simulink model "ejh44b"  (Simulink 3.00)
settings: Solver=ode45  StartTime=0.0  StopTime=10.0  RelTol=1e-3
settings Model: LastModifiedBy=Administrador

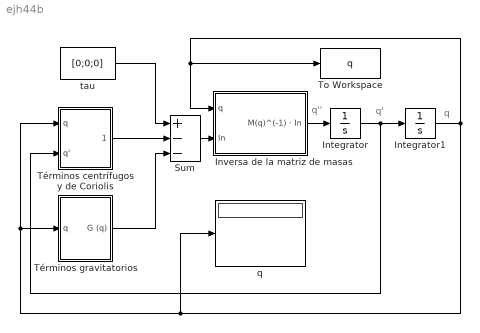
== system ejh44b ==
  note: q'
  note: q''
  note: q
  Integrator : Integrator  ExternalReset=none  InitialConditionSource=internal  InitialCondition=[0;0;0]  LimitOutput=off  UpperSaturationLimit=inf  LowerSaturationLimit=-inf  ShowSaturationPort=off  ShowStatePort=off  AbsoluteTolerance=auto
  Integrator1 : Integrator  ExternalReset=none  InitialConditionSource=internal  InitialCondition=[pi/6; pi/6; pi/18]  LimitOutput=off  UpperSaturationLimit=inf  LowerSaturationLimit=-inf  ShowSaturationPort=off  ShowStatePort=off  AbsoluteTolerance=auto
  Inversa de la matriz de masas : Subsystem  mask(Término de Coriolis){dyn=[0 0 0 0 0 4.7 0.8 0 0 0 0 0 0 0 0 0 1 0 0 0;0 0.8 0 0 0 2.6 0.8 0 0 0 0 0 0 0 0 0 1 0 0 0;0 0.8 0 0 0 1.1 0 0 0 0.05 0.1 0.1 0 0 0 0 1 0 0 0]}
      mask prompts: dyn "Matriz de parámetros dinámicos:"
      mask help: Este bloque devuelve el par correspondiente al término de Coriolis.
      mask Help: A este bloque hay que darle tres parámetros: 1) La matriz de parámetros dinámicos del manipulador de acuerdo con el formato que se explica en la sección "dyn" del Apéndice, 2) Un vector columna correspondiente a la aceleración de la gravedad, y 3) Un vector columna correspondiente a las fuerzas externas.
  Sum : Sum  Inputs=+--  SaturateOnIntegerOverflow=on
  To Workspace : ToWorkspace  VariableName=q  SampleTime=-1  SaveFormat=Matrix
  Términos gravitatorios : Subsystem  mask(Término gravitatorio){dyn=[0 0 0 0 0 4.7 0.8 0 0 0 0 0 0 0 0 0 1 0 0 0;0 0.8 0 0 0 2.6 0.8 0 0 0 0 0 0 0 0 0 1 0 0 0;0 0.8 0 0 0 1.1 0 0 0 0.05 0.1 0.1 0 0 0 0 1 0 0 0], grav=[0 -9.8 0]}
      mask prompts: dyn "Matriz de parámetros cinemáticos y dinámicos:"; grav "Vector aceleración de la gravedad:"
      mask help: Este bloque calcula el par correspondiente al término gravitatorio.
  Términos centrífugos y de Coriolis : Subsystem  mask(Término de Coriolis){dyn=[0 0 0 0 0 4.7 0.8 0 0 0 0 0 0 0 0 0 1 0 0 0;0 0.8 0 0 0 2.6 0.8 0 0 0 0 0 0 0 0 0 1 0 0 0;0 0.8 0 0 0 1.1 0 0 0 0.05 0.1 0.1 0 0 0 0 1 0 0 0]}
      mask prompts: dyn "Matriz de parámetros dinámicos:"
      mask help: Este bloque devuelve el par correspondiente al término de Coriolis.
      mask Help: A este bloque hay que darle tres parámetros: 1) La matriz de parámetros dinámicos del manipulador de acuerdo con el formato que se explica en la sección "dyn" del Apéndice, 2) Un vector columna correspondiente a la aceleración de la gravedad, y 3) Un vector columna correspondiente a las fuerzas externas.
  q : Display
      settings: Format=short
  tau : Constant  Value=[0;0;0]
  wires:
  Términos centrífugos y de Coriolis/1(V (q,q')) -> Sum/2
  Sum/1 -> Inversa de la matriz de masas/2(In)
  Inversa de la matriz de masas/1(M(q)^(-1) · In) -> Integrator/1
  Integrator/1 -> Integrator1/1, Términos centrífugos y de Coriolis/2(q')
  Integrator1/1 -> Inversa de la matriz de masas/1(q), To Workspace/1, Términos centrífugos y de Coriolis/1(q), Términos gravitatorios/1(q), q/1
  Términos gravitatorios/1(G (q)) -> Sum/3
  tau/1 -> Sum/1

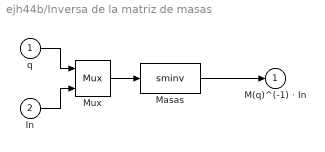
== system ejh44b/Inversa de la matriz de masas ==
  q : Inport  Port=1  PortWidth=-1  SampleTime=-1  DataType=auto
      settings: SignalType=auto
  In : Inport  Port=2  PortWidth=-1  SampleTime=-1  DataType=auto
      settings: SignalType=auto
  Masas : S-Function  FunctionName=sminv  Parameters=dyn  PortCounts=[]  SFunctionModules=''
  Mux : Mux  Inputs=2
      settings: DisplayOption=none
  M(q)^(-1) · In : Outport  Port=1  InitialOutput=0
  wires:
  Masas/1 -> M(q)^(-1) · In/1
  In/1 -> Mux/2
  q/1 -> Mux/1
  Mux/1 -> Masas/1

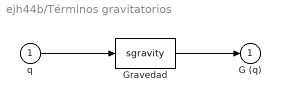
== system ejh44b/Términos gravitatorios ==
  q : Inport  Port=1  PortWidth=-1  SampleTime=-1  DataType=auto
      settings: SignalType=auto
  Gravedad : S-Function  FunctionName=sgravity  Parameters=dyn,grav  PortCounts=[]  SFunctionModules=''
  G (q) : Outport  Port=1  InitialOutput=0
  wires:
  q/1 -> Gravedad/1
  Gravedad/1 -> G (q)/1

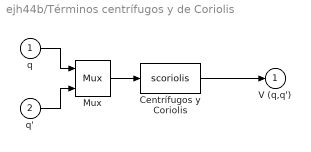
== system ejh44b/Términos centrífugos y de Coriolis ==
  q : Inport  Port=1  PortWidth=-1  SampleTime=-1  DataType=auto
      settings: SignalType=auto
  q' : Inport  Port=2  PortWidth=-1  SampleTime=-1  DataType=auto
      settings: SignalType=auto
  Centrífugos y Coriolis : S-Function  FunctionName=scoriolis  Parameters=dyn  PortCounts=[]  SFunctionModules=''
  Mux : Mux  Inputs=2
      settings: DisplayOption=none
  V (q,q') : Outport  Port=1  InitialOutput=0
  wires:
  Centrífugos y Coriolis/1 -> V (q,q')/1
  q'/1 -> Mux/2
  q/1 -> Mux/1
  Mux/1 -> Centrífugos y Coriolis/1
